simulink model "pitch_only"  (R2022a)
settings: Solver=VariableStepAuto  StartTime=0.0  StopTime=10.0  RelTol=1e-3
values from neighbouring files (symbols this model uses):
  A_p = [0,1;0,0]    [pitch_experi.m]    (also in pitch_ref.m)
  B_p = [0,0;0,0.248000000000000]    [pitch_experi.m]    (also in pitch_ref.m = [0,0;0,21.6319])
  C_p = [1,0]    [pitch_experi.m]    (also in pitch_ref.m = [1,0;0,1])
  D_p = [0,0]    [pitch_experi.m]    (also in pitch_ref.m = [0,0;0,0])
libraries: mpclib x1
settings Model: Creator=s615g  LastModifiedBy=s615g

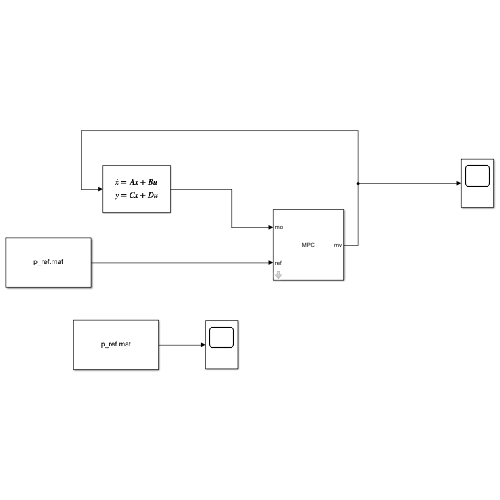
[thumbnail: Simulink's stored preview of the top-level diagram]
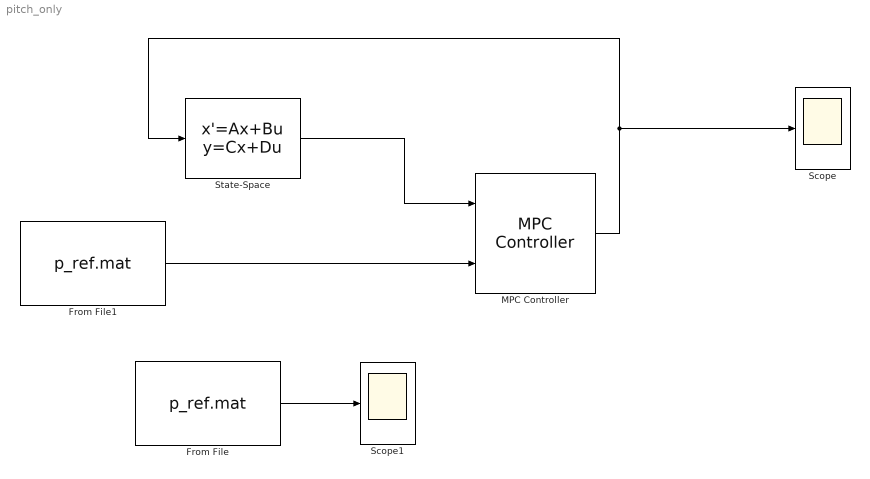
== system pitch_only ==
  From File : FromFile  FileName=p_ref.mat  SampleTime=0
  From File1 : FromFile  FileName=p_ref.mat  SampleTime=0
  MPC Controller : mpclib/MPC Controller  SCDEnableBlockLinearizationSpecification=on  is_multiple=0  enable_value=0  return_u0=off  updateMPCinCallerWorkspace=on  md_inport=off  mv_inport=off  uref_inport=off  return_cost=off  return_mvseq=off  return_qpstatus=off  return_xseq=off  return_state=off  return_ovseq=off  state_inport=off  umin_inport=off  umax_inport=off  ymin_inport=off  ymax_inport=off  cc_inport=off  ywt_inport=off  uwt_inport=off  duwt_inport=off  rhoeps_inport=off  pm_inport=off  MaximumP=10  HorizonChoice=FixedHorizon  n_ts=1  n_p=10  n_mv=1  n_md=1  n_ud=0  n_mo=1  n_uo=0  BlockDataType=double  SampleTimeInherited=off  switch_inport=off
  Scope : Scope
  Scope1 : Scope
  State-Space : StateSpace  A=A_p  B=B_p  C=C_p  D=D_p  InitialCondition=0  ParameterTunability=Unconstrained  AllowTunableDMatrix=on
  wires:
  From File1/1 -> MPC Controller/2
  State-Space/1 -> MPC Controller/1
  MPC Controller/1 -> State-Space/1, Scope/1
  From File/1 -> Scope1/1
